simulink model "EKF_Pose_estimation"  (R2020b)
settings: Solver=FixedStepDiscrete  StartTime=0.0  StopTime=60  FixedStep=0.02  RelTol=1e-3  EnableMultiTasking=on
InitFcn:
  | load('Encoder_Data.mat')
  | ProcNoiseD=0.03^2; % is a variance
  | ProcNoiseTheta=0.009^2; % is a variance
  | Ts=0.02
StopFcn:
  | I = imread('Enviroment.png');
  | x = [0 35.9];
  | y=[23.31 0];
  | image(I,'XData',x,'YData',y);
  | axis xy;
  | hold on
  | plot (Pose_t.Data(:,1),Pose_t.Data(:,2),'b');
  | plot (Pose_est.Data(:,1),Pose_est.Data(:,2),'r');
  | len=length(Pose_t.Data);
  | for i=1:round(len/15):len
  | %    plot_ellipse(Pk.signals.values(1:2,1:2,i),[xEst.signals.values(i,1), xEst.signals.values(i,2)],'g');
  |     plot_ellipse(Pk.signals.values(1:2,1:2,i),[Pose_est.Data(i,1), Pose_est.Data(i,2)],'g');
  |     title(' EKF Pose stimated');
  | end
settings Model: Creator=antonio  LastModifiedBy=antonio
settings DataIOCC: LimitDataPoints=on  SaveFormat=Array  ReturnWorkspaceOutputs=off
settings OptimizationCC: LifeSpan=inf
settings DebuggingCC: UnderspecifiedInitializationDetection=Classic  MergeDetectMultiDrivingBlocksExec=none  SolverPrmCheckMsg=warning  StateNameClashWarn=warning  SFUnexpectedBacktrackingDiag=warning  SFNoUnconditionalDefaultTransitionDiag=warning  SFExecutionAtInitializationDiag=none  ArithmeticOperatorsInVariantConditions=warning
settings HardwareCC: ProdBitPerPointer=32  ProdBitPerSizeT=32  ProdBitPerPtrDiffT=32  ProdLargestAtomicFloat=None  ProdIntDivRoundTo=Undefined  ProdEndianess=Unspecified  ProdWordSize=32  ProdHWDeviceType=32-bit Generic
settings ModelReferenceCC: PropagateSignalLabelsOutOfModel=off
settings SFSimCC: SimUseLocalCustomCode=off  CustomCodeUndefinedFunction=UseInterfaceOnly
settings RTWCC: RTWUseLocalCustomCode=off
settings CodeAppCC: StateflowObjectComments=on
settings GRTTargetCC: TargetLangStandard=C89/C90 (ANSI)
settings ConfigComp: CovMetricSettings=dw  CovSaveCumulativeToWorkspaceVar=on  CovSaveSingleToWorkspaceVar=on  CovExternalEMLEnable=off

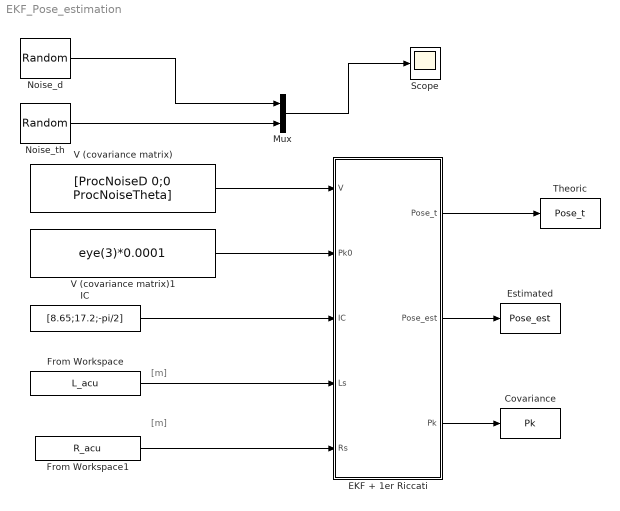
== system EKF_Pose_estimation ==
  note: [m]
  note: [m]
  Covariance : ToWorkspace  VariableName=Pk  SaveFormat=Structure With Time  SampleTime=-1
  EKF + 1er Riccati : MATLAB Function  TreatAsAtomicUnit=on
  Estimated : ToWorkspace  VariableName=Pose_est  SaveFormat=Timeseries  SampleTime=-1
  From Workspace : FromWorkspace  VariableName=L_acu  SampleTime=Ts
  From Workspace1 : FromWorkspace  VariableName=R_acu
  IC : Constant  Value=[8.65;17.2;-pi/2]
  Mux : Mux  Inputs=2
  Noise_d : RandomNumber  Variance=ProcNoiseD  Seed=2
  Noise_th : RandomNumber  Variance=ProcNoiseTheta  Seed=2
  Scope : Scope
  Theoric : ToWorkspace  VariableName=Pose_t  SaveFormat=Timeseries  SampleTime=-1
  V (covariance matrix) : Constant  Value=[ProcNoiseD 0;0 ProcNoiseTheta]  VectorParams1D=off
  V (covariance matrix)1 : Constant  Value=eye(3)*0.0001  VectorParams1D=off
  wires:
  IC/1 -> EKF + 1er Riccati/3(IC)
  EKF + 1er Riccati/1(Pose_t) -> Theoric/1
  EKF + 1er Riccati/2(Pose_est) -> Estimated/1
  From Workspace1/1 -> EKF + 1er Riccati/5(Rs)
  From Workspace/1 -> EKF + 1er Riccati/4(Ls)
  V (covariance matrix)1/1 -> EKF + 1er Riccati/2(Pk0)
  EKF + 1er Riccati/3(Pk) -> Covariance/1
  Noise_d/1 -> Mux/1
  Noise_th/1 -> Mux/2
  V (covariance matrix)/1 -> EKF + 1er Riccati/1(V)
  Mux/1 -> Scope/1

== matlab function EKF_Pose_estimation/EKF + 1er Riccati ==
  data: V input; Pk0 input; Pose_t output; Pose_est output; IC input; Ls input; Rs input; Pk output
function [Pose_t,Pose_est,Pk] = fcn(V,Pk0,IC,Ls,Rs) % IC->Initial Condition [xo,yo,th0]
                                   % R and L are the displacements of
                                   % wheels [m]
persistent L_ant R_ant...
           x_w y_w suma_theta...%  internal variable to be mantain its values
           x_w_est y_w_est suma_theta_est...%  internal variable to be mantain its values
           Pose_est1 Pk1

ts=0.02; % sample time
S = 0.26;

%%%%%%%%%%%%%%%%%%%%%%%%%%%%%%%%%%%%%%%%%%%%%%%%%%%%%%%%%%%%%%%%%%%%%%%%%%
% %%%%%%%%%%%%%%   Read Initial condition   %%%%%%%%%%%%%%%%%%%%%%%%%%%%%%
x_ini=IC(1);
y_ini=IC(2);
theta_ini=IC(3);
P_ini=Pk0;
%%%%%%%%%%%%%%%%%%%%%%%%%%%%%%%%%%%%%%%%%%%%%%%%%%%%%%%%%%%%%%%%%%%%%%%%%%
%%%%%%%%%%%%%%%   variable initialitation  %%%%%%%%%%%%%%%%%%%%%%%%%%%%%%
if isempty (x_w)
    L_ant=0;
    R_ant=0;
    x_w=x_ini;
    y_w=y_ini;
    suma_theta=theta_ini; 
    x_w_est=x_ini;
    y_w_est=y_ini;
    suma_theta_est=theta_ini; 
    
    
    Pose_est1 = [x_w;y_w;suma_theta];
    Pose_t=[x_w;y_w;suma_theta];
    Pk1 = P_ini;
end

%%%%%%%%%%%%%%%%%%%%%%%%%%%%%%%%%%%%%%%%%%%%%%%%%%%%%%%%%%%%%%%%%%%%%%%%%
%%%%%%%%%%%%%%%%%  Compute R_inc & L_inc   %%%%%%%%%%%%%%%%%%%%%%%%%%%%%%
R=Rs-R_ant;
L=Ls-L_ant;
R_ant=Rs;
L_ant=Ls;

%%%%%%%%%%%%%%%%%%%%%%%%%%%%%%%%%%%%%%%%%%%%%%%%%%%%%%%%%%%%%%%%%%%%%%%%%%
%%%%%%%%%%%%%%%%%  Compute the odometry    %%%%%%%%%%%%%%%%%%%%%%%%%%%%%%%
delta_th = ((R-L)/(2*S));
delta_d = (R+L)/2;
%%%%%%%%%%%%%%%%%%%%%%%%%%%%%%%%%%%%%%%%%%%%%%%%%%%%%%%%%%%%%%%%%%%%%%%%%%
%%%%%%%%%%%%%%%%%  integration of the robot pose %%%%%%%%%%%%%%%%%%%%%%%%%%
suma_theta=mod((suma_theta+delta_th),2*pi);
x_w = x_w + delta_d *cos(suma_theta);
y_w = y_w + delta_d *sin(suma_theta);
Pose_t=[x_w;y_w;suma_theta];

%%%%%%%%%%%%%%%%%%%%%%%%%%%%%%%%%%%%%%%%%%%%%%%%%%%%%%%%%%%%%%%%%%%%%%%%%%
%%%%%%%%%%%%%%%%%  Build the Jacocian %%%%%%%%%%%%%%%%%%%%%%%%%%%%%%%%%%%%3

F_x = [1 0 -delta_d*sin(suma_theta);....
       0 1  delta_d*cos(suma_theta);....
       0 0 1];

F_v = [cos(suma_theta) 0;....
       sin(suma_theta) 0;...
       0 1];

%%%%%%%%%%%%%%%%%%%%%%%%%%%%%%%%%%%%%%%%%%%%%%%%%%%%%%%%%%%%%%%%%%%%%%%%%%
%%%%%%%%%%%%%%%%% Compute the EKF Trucated Taylor %%%%%%%%%%%%%%%%%%%%%%%%
%randinit;
n_d=rand*V(1,1)
n_th=rand*V(2,2)
suma_theta_est=mod((suma_theta_est+delta_th+n_th),2*pi);
x_w_est = x_w_est + (delta_d+n_d)*cos(suma_theta_est);
y_w_est = y_w_est + (delta_d+n_d) *sin(suma_theta_est);
Pose_est1=[x_w_est;y_w_est;suma_theta_est];

%Pose_est1 = Pose_est1 + F_x*(Pose_t - Pose_est1) + F_v*[V(1);V(2)];
%Pose_est1 = F_x*(Pose_est1) + F_v*diag(V);

Pk1 = F_x*Pk1*F_x' + F_v*[V(1) 0;0 V(2)]*F_v';

%%%%%%%%%%%%%%%%%%%%%%%%%%%%%%%%%%%%%%%%%%%%%%%%%%%%%%%%%%%%%%%%%%%%%%%%%%
%%%%%%%%%%%%%%%%%  output variable %%%%%%%%%%%%%%%%%%%%%%%%%%%%%%%%%%%%%%%

Pose_t=[x_w;y_w;suma_theta]
Pose_est= Pose_est1
Pk=Pk1

end
